simulink library "Lib_EMTAT"  (R2021b)
settings: Solver=VariableStepAuto  StartTime=0.0  StopTime=10.0  RelTol=1e-3
undefined symbols (not defined in the file or in its folder): A_M, B_M, Cj, component_degradation_input, Cs, E0_M, f_sw, K_M, MWS, Q_M, Q_rr, r_c, r_D, R_M, Rj, Ru, SNR_DX_M, SNR_IC_M, SNR_Mn_M, SNR_Mx_M, SOC_Init_M, u_ce0, u_D0
libraries: $bdroot x82, simulink x23, Lib_Dyn_StateSpace_EMTAT x3, PB_Library_Master_Working x1
(part 6 of 7)

== system Lib_EMTAT/Components/Physics-Based/Motor /Torque Saturation Logic ==
  note: Needs: P_m_max, T_ref_max
  T_ref_in : Inport
  S : Inport  Port=2
  Abs : Abs
  Constant1 : Constant  Value=P_out_max
  Display : Display
  Display1 : Display
  Display2 : Display
  Divide : Product  Inputs=*/
  Product : Product
  Sat in ft-lbs : Saturate  UpperLimit=T_nom  LowerLimit=-T_nom
  Switch : Switch  Criteria=u2 > Threshold  Threshold=P_out_max
  ft-lbs to Nm : Gain  Gain=1.3558
  ft-lbs to Nm1 : Gain  Gain=1.3558
  T_ref_sat : Outport  VectorParamsAs1DForOutWhenUnconnected=off
  wires:
  T_ref_in/1 -> Sat in ft-lbs/1, ft-lbs to Nm/1  "ft-lbs"
  Constant1/1 -> Display/1, Divide/1  "W"
  S/1 -> Product/2, Divide/2
  Sat in ft-lbs/1 -> ft-lbs to Nm1/1
  Product/1 -> Abs/1  "W"
  Switch/1 -> T_ref_sat/1
  ft-lbs to Nm/1 -> Product/1
  ft-lbs to Nm1/1 -> Switch/3, Display1/1  "Nm"
  Abs/1 -> Display2/1, Switch/2
  Divide/1 -> Switch/1  "Nm"

== system Lib_EMTAT/Components/Physics-Based/Motor /Vdq ==
  Id : Inport
  w_elec : Inport  Port=2
  Iq : Inport  Port=3
  Res_DF : Inport  Port=4
  Flux_DF : Inport  Port=5
  Divide : Product  Inputs=/*
  Divide1 : Product  Inputs=*/
  Gain : Gain  Gain=R_s
  Gain1 : Gain  Gain=R_s
  Gain2 : Gain  Gain=L_s
  Gain3 : Gain  Gain=flux_m
  Product : Product
  Product1 : Product
  Product2 : Product
  Subtract : Sum  Inputs=+-
  Sum : Sum  Inputs=+++
  Vd : Outport  VectorParamsAs1DForOutWhenUnconnected=off
  Vq : Outport  Port=2  VectorParamsAs1DForOutWhenUnconnected=off
  wires:
  Id/1 -> Product1/1, Gain/1
  Iq/1 -> Gain1/1, Product/2
  w_elec/1 -> Gain3/1, Gain2/1
  Gain2/1 -> Product/1, Product1/2
  Product/1 -> Subtract/2
  Subtract/1 -> Vd/1
  Product1/1 -> Sum/1
  Sum/1 -> Vq/1
  Gain3/1 -> Product2/1
  Product2/1 -> Sum/3
  Flux_DF/1 -> Product2/2
  Divide/1 -> Subtract/1
  Gain/1 -> Divide/2
  Res_DF/1 -> Divide/1, Divide1/2
  Divide1/1 -> Sum/2
  Gain1/1 -> Divide1/1

== system Lib_EMTAT/Components/Physics-Based/Motor /Vs ==
  Vd : Inport
  Vq : Inport  Port=2
  Add : Sum
  Square : Math  Operator=square  SignedPower=on  SaturateOnIntegerOverflow=on
  Square Root : Sqrt  SaturateOnIntegerOverflow=on
  Square1 : Math  Operator=square  SignedPower=on  SaturateOnIntegerOverflow=on
  Vs : Outport  VectorParamsAs1DForOutWhenUnconnected=off
  wires:
  Vq/1 -> Square/1
  Vd/1 -> Square1/1
  Square1/1 -> Add/1
  Square/1 -> Add/2
  Add/1 -> Square Root/1
  Square Root/1 -> Vs/1

== system Lib_EMTAT/Components/Physics-Based/Rectifier/Diode Conduction Losses1 ==
  note: update with gradual degredation term later
  note: the aDF must increase u_D_M
  note: You need to read from graphs:
      |
      | -U_ce0
      | -Rc=dU_ce/dI_c (linear)
      | -U_D0
      | -R_D=dU_D/dI_D (linear)
  I_M : Inport
  PF : Inport  Port=2
  m : Inport  Port=3
  T : Inport  Port=4
  1-D Lookup Table r_D : Lookup_n-D  NumberOfTableDimensions=1  BreakpointsForDimension1=T_M  Table=R_D_M  InternalRulePriority=Speed  RndMeth=Simplest  InputSameDT=on
  1-D Lookup Table u_D0 : Lookup_n-D  NumberOfTableDimensions=1  BreakpointsForDimension1=T_M  Table=u_D_M  InternalRulePriority=Speed  RndMeth=Simplest  InputSameDT=on
  Constant : Constant  Value=1/(2*pi)
  Constant1 : Constant  Value=1/8
  Gain : Gain  Commented=on  Gain=u_D0
  Gain1 : Gain  Gain=1/8
  Gain2 : Gain  Commented=on  Gain=r_D
  Gain3 : Gain  Gain=1/(3*pi)
  Product{,1..4} (5 alike) : Product
  Square : Math  Operator=square  SignedPower=on  SaturateOnIntegerOverflow=on
  Sum : Sum  Inputs=+-
  Sum2 : Sum
  Sum3 : Sum  Inputs=-+
  P_CD : Outport  VectorParamsAs1DForOutWhenUnconnected=off
  wires:
  1-D Lookup Table r_D/1 -> Product4/2
  1-D Lookup Table u_D0/1 -> Product3/2
  T/1 -> 1-D Lookup Table r_D/1, 1-D Lookup Table u_D0/1
  Sum3/1 -> Product2/2
  Constant1/1 -> Sum3/2
  Product4/1 -> Product2/1
  Gain3/1 -> Sum3/1
  Square/1 -> Product4/1
  Sum/1 -> Product/1
  Product1/1 -> Gain1/1, Gain3/1
  Gain1/1 -> Sum/2
  m/1 -> Product1/2
  PF/1 -> Product1/1
  Constant/1 -> Sum/1
  Product3/1 -> Square/1, Product/2
  I_M/1 -> Product3/1  "I_M"
  Sum2/1 -> P_CD/1
  Product2/1 -> Sum2/2
  Product/1 -> Sum2/1

== system Lib_EMTAT/Components/Physics-Based/Rectifier/IGBT Conduction Losses1 ==
  note: You need to read from graphs:
      |
      | -U_ce0
      | -Rc=dU_ce/dI_c (linear)
      | -U_D0
      | -R_D=dU_D/dI_D (linear)
  I_M : Inport
  PF : Inport  Port=2
  m : Inport  Port=3
  T : Inport  Port=4
  1-D Lookup Table r_c : Lookup_n-D  NumberOfTableDimensions=1  BreakpointsForDimension1=T_M  Table=R_c_M  InternalRulePriority=Speed  RndMeth=Simplest  InputSameDT=on
  1-D Lookup Table u_ce0 : Lookup_n-D  NumberOfTableDimensions=1  BreakpointsForDimension1=T_M  Table=u_ce0_M  InternalRulePriority=Speed  RndMeth=Simplest  InputSameDT=on
  Constant : Constant  Value=1/(2*pi)
  Constant1 : Constant  Value=1/8
  Gain : Gain  Commented=on  Gain=u_ce0
  Gain1 : Gain  Gain=1/8
  Gain2 : Gain  Commented=on  Gain=r_c
  Gain3 : Gain  Gain=1/(3*pi)
  Product{,1..4} (5 alike) : Product
  Square : Math  Operator=square  SignedPower=on  SaturateOnIntegerOverflow=on
  Sum : Sum
  Sum2 : Sum
  Sum3 : Sum
  P_CT : Outport  VectorParamsAs1DForOutWhenUnconnected=off
  wires:
  1-D Lookup Table r_c/1 -> Product4/2
  1-D Lookup Table u_ce0/1 -> Product3/2
  T/1 -> 1-D Lookup Table r_c/1, 1-D Lookup Table u_ce0/1
  Sum3/1 -> Product2/2
  Constant1/1 -> Sum3/2
  Product4/1 -> Product2/1
  Gain3/1 -> Sum3/1
  Square/1 -> Product4/1
  Sum/1 -> Product/1
  Product1/1 -> Gain1/1, Gain3/1
  Gain1/1 -> Sum/2
  m/1 -> Product1/2
  PF/1 -> Product1/1
  Constant/1 -> Sum/1
  Product3/1 -> Square/1, Product/2
  I_M/1 -> Product3/1  "I_M"
  Sum2/1 -> P_CT/1
  Product2/1 -> Sum2/2
  Product/1 -> Sum2/1

== system Lib_EMTAT/Components/Physics-Based/Rectifier/IGBT Switching Losses1 ==
  note: the aDF must increase E1_M
  note: update with gradual degredation term later
  I_ce : Inport
  T : Inport  Port=2
  1-D Lookup Table E0 : Lookup_n-D  NumberOfTableDimensions=1  BreakpointsForDimension1=T_M  Table=E0_M  InternalRulePriority=Speed  RndMeth=Simplest  InputSameDT=on
  1-D Lookup Table E1 : Lookup_n-D  NumberOfTableDimensions=1  BreakpointsForDimension1=T_M  Table=E1_M  InternalRulePriority=Speed  RndMeth=Simplest  InputSameDT=on
  Add : Sum
  Constant : Constant  Value=f_sw_M
  Constant1 : Constant
  Divide : Product  Inputs=*/
  Product : Product
  Product1 : Product
  P_ST : Outport  VectorParamsAs1DForOutWhenUnconnected=off
  wires:
  Product/1 -> P_ST/1
  Add/1 -> Product/1
  I_ce/1 -> Product1/1
  1-D Lookup Table E0/1 -> Add/1
  Product1/1 -> Add/2
  T/1 -> 1-D Lookup Table E0/1, 1-D Lookup Table E1/1
  1-D Lookup Table E1/1 -> Product1/2
  Constant/1 -> Divide/1
  Divide/1 -> Product/2
  Constant1/1 -> Divide/2

== system Lib_EMTAT/Components/Physics-Based/Rectifier/I_Ripple1 ==
  note: update with gradual degredation term later
  V_batt : Inport
  "V_M " : Inport  Port=2
  Constant : Constant  Value=L_s_M
  Constant1 : Constant
  Divide : Product  Inputs=*/
  Divide1 : Product  Inputs=*/
  Gain : Gain  Gain=sqrt(2)
  Gain1 : Gain  Gain=2
  Gain2 : Gain  Gain=f_sw_M
  Product : Product
  Product1 : Product
  Subtract : Sum  Inputs=+-
  I_Rip : Outport  VectorParamsAs1DForOutWhenUnconnected=off
  wires:
  Divide/1 -> I_Rip/1
  Product1/1 -> Gain2/1
  Gain1/1 -> Product1/2
  Constant/1 -> Gain1/1
  Product/1 -> Divide/1
  Subtract/1 -> Product/1
  V_batt/1 -> Product1/1, Subtract/1
  Gain/1 -> Subtract/2
  "V_M "/1 -> Gain/1, Product/2
  Gain2/1 -> Divide1/1
  Constant1/1 -> Divide1/2
  Divide1/1 -> Divide/2

== system Lib_EMTAT/Components/Physics-Based/Rectifier/P_out_gen ==
  I (DC) : Inport
  V_s (DC) : Inport  Port=2
  PF : Inport  Port=3
  Display : Display
  Gain : Gain  Commented=through  Gain=sqrt(3)
  PowerFactor StandIn : Constant
  Product : Product  Inputs=3
  P_out_gen : Outport  VectorParamsAs1DForOutWhenUnconnected=off
  wires:
  PowerFactor StandIn/1 -> Product/3
  Product/1 -> Gain/1
  Gain/1 -> P_out_gen/1
  V_s (DC)/1 -> Product/1
  PF/1 -> Display/1
  I (DC)/1 -> Product/2

== system Lib_EMTAT/Components/Physics-Based/Rectifier/mVal ==
  V_s : Inport
  V_batt : Inport  Port=2
  Divide : Product  Inputs=*/
  Gain : Gain  Gain=sqrt(2)
  m : Outport  VectorParamsAs1DForOutWhenUnconnected=off
  wires:
  V_batt/1 -> Divide/2
  Gain/1 -> Divide/1
  V_s/1 -> Gain/1
  Divide/1 -> m/1

== system Lib_EMTAT/Components/Power Flow/AC-AC Transformer/Compensate for Divide By Zero ==
  note: If Vin is not equal to zero, use its value.
      | If Vin is equal to zero, it will calculate a nan value for Iin. Set Iin to zero.
  P_AC_1 : Inport
  V_LN_rms_1 : Inport  Port=2
  Fix Divide By Zero. : Subsystem
  I_L_rms_1 : Outport
  wires:
  V_LN_rms_1/1 -> Fix Divide By Zero./1(V_LN_rms_1)
  P_AC_1/1 -> Fix Divide By Zero./2(P_AC_1)
  Fix Divide By Zero./1(I_L_rms_1) -> I_L_rms_1/1

== system Lib_EMTAT/Components/Power Flow/AC-AC Transformer/Direction Determination ==
  P_AC_2 : Inport
  Ploss : Inport  Port=2
  Add1 : Sum
  Switch : Switch  Criteria=u2 ~= 0
  P_AC_1 : Outport
  wires:
  Add1/1 -> Switch/1
  Switch/1 -> P_AC_1/1
  P_AC_2/1 -> Switch/2, Switch/3, Add1/2
  Ploss/1 -> Add1/1

== system Lib_EMTAT/Components/Power Flow/AC-AC Transformer/Efficiency ==
  P_AC_2 : Inport
  P_AC_1 : Inport  Port=2
  Abs : Abs
  Abs1 : Abs
  Fix Divide By Zero. : Subsystem
  Fix Divide By Zero.1 : Subsystem
  GreaterThan : RelationalOperator  OutDataTypeStr=boolean  RndMeth=Simplest
  Switch : Switch  Criteria=u2 > Threshold
  Eff : Outport
  wires:
  Switch/1 -> Eff/1
  GreaterThan/1 -> Switch/2
  Abs1/1 -> Fix Divide By Zero.1/2(abs(P_AC_2)), Fix Divide By Zero./1(abs(P_AC_2)), GreaterThan/2
  P_AC_1/1 -> Abs/1
  P_AC_2/1 -> Abs1/1
  Abs/1 -> Fix Divide By Zero.1/1(abs(P_AC_1)), Fix Divide By Zero./2(abs(P_AC_1)), GreaterThan/1
  Fix Divide By Zero./1(Eff) -> Switch/3
  Fix Divide By Zero.1/1(Eff) -> Switch/1

== system Lib_EMTAT/Components/Power Flow/AC-AC Transformer/Failure Determination ==
  Fail? : Inport
  Compare To Constant : simulink/Logic and Bit Operations/Compare To Constant  relop===  const=1  OutDataTypeStr=boolean
  Compare To Constant1 : simulink/Logic and Bit Operations/Compare To Constant  relop===  const=2  OutDataTypeStr=boolean
  Data Type Conversion : DataTypeConversion  OutDataTypeStr=double
  Data Type Conversion1 : DataTypeConversion  OutDataTypeStr=double
  Failure Mode : Constant  Value=FM
  Logical Operator : Logic  AllPortsSameDT=off  OutDataTypeStr=boolean
  Logical Operator1 : Logic  AllPortsSameDT=off  OutDataTypeStr=boolean
  OCFail : Outport
  DegFail : Outport  Port=2
  wires:
  Failure Mode/1 -> Compare To Constant1/1, Compare To Constant/1
  Compare To Constant/1 -> Logical Operator/1
  Logical Operator/1 -> Data Type Conversion/1
  Compare To Constant1/1 -> Logical Operator1/1
  Logical Operator1/1 -> Data Type Conversion1/1
  Fail?/1 -> Logical Operator1/2, Logical Operator/2
  Data Type Conversion1/1 -> DegFail/1
  Data Type Conversion/1 -> OCFail/1

== system Lib_EMTAT/Components/Power Flow/AC-AC Transformer/Open Circuit Failure - DC Current ==
  Failed? : Inport
  I_L_rms_1 : Inport  Port=2
  Constant : Constant  Value=0
  IsInf : RelationalOperator  Operator=isInf  OutDataTypeStr=boolean  RndMeth=Simplest
  IsNaN : RelationalOperator  Operator=isNaN  OutDataTypeStr=boolean  RndMeth=Simplest
  Logical Operator : Logic  Operator=OR  Inputs=3  AllPortsSameDT=off  OutDataTypeStr=boolean
  Switch : Switch  Criteria=u2 > Threshold
  "I_L_rms_1 " : Outport
  wires:
  Failed?/1 -> Logical Operator/1
  Constant/1 -> Switch/1
  I_L_rms_1/1 -> IsNaN/1, IsInf/1, Switch/3
  Switch/1 -> "I_L_rms_1 "/1
  Logical Operator/1 -> Switch/2
  IsNaN/1 -> Logical Operator/2
  IsInf/1 -> Logical Operator/3

== system Lib_EMTAT/Components/Power Flow/AC-AC Transformer/Open Circuit Failure - Line to Neutral Voltage ==
  Failed? : Inport
  V_LN_rms_2 : Inport  Port=2
  Constant : Constant  Value=0
  IsInf : RelationalOperator  Operator=isInf  OutDataTypeStr=boolean  RndMeth=Simplest
  IsNaN : RelationalOperator  Operator=isNaN  OutDataTypeStr=boolean  RndMeth=Simplest
  Logical Operator : Logic  Operator=OR  Inputs=3  AllPortsSameDT=off  OutDataTypeStr=boolean
  Switch : Switch  Criteria=u2 > Threshold
  "V_LN_rms_2 " : Outport
  wires:
  IsInf/1 -> Logical Operator/3
  IsNaN/1 -> Logical Operator/2
  Logical Operator/1 -> Switch/2
  Switch/1 -> "V_LN_rms_2 "/1
  V_LN_rms_2/1 -> Switch/3, IsInf/1, IsNaN/1
  Constant/1 -> Switch/1
  Failed?/1 -> Logical Operator/1

== system Lib_EMTAT/Components/Power Flow/AC-AC Transformer/Open Circuit// Degradation Failure ==
  Ploss : Inport
  DegFail? : Inport  Port=2
  OCFail? : Inport  Port=3
  Deg : Inport  Port=4
  Constant : Constant  Value=0
  Constant1 : Constant  Value=Plosslim
  Divide : Product  Inputs=**
  "If degradation failure, add to Ploss." : Switch  Criteria=u2 > Threshold
  "If open circuit failure, set Ploss = 0." : Switch  Criteria=u2 > Threshold
  Sum1 : Sum  Inputs=++|
  "Ploss " : Outport
  wires:
  DegFail?/1 -> "If degradation failure, add to Ploss."/2
  "If degradation failure, add to Ploss."/1 -> "If open circuit failure, set Ploss = 0."/3
  Ploss/1 -> Sum1/2, "If degradation failure, add to Ploss."/3
  Sum1/1 -> "If degradation failure, add to Ploss."/1
  Deg/1 -> Divide/2
  "If open circuit failure, set Ploss = 0."/1 -> "Ploss "/1
  OCFail?/1 -> "If open circuit failure, set Ploss = 0."/2
  Constant/1 -> "If open circuit failure, set Ploss = 0."/1
  Constant1/1 -> Divide/1
  Divide/1 -> Sum1/1

== system Lib_EMTAT/Components/Power Flow/AC-AC Transformer/Power Loss ==
  V_LN_rms_1 : Inport
  I_L_rms_2 : Inport  Port=2
  2-D Lookup Table : Lookup_n-D  BreakpointsForDimension1=X_C_VoltageAC1Vec_M  BreakpointsForDimension2=Y_C_CurrentAC2Vec_M  Table=T_C_PowLossArray_M  ExtrapMethod=Clip  UseLastTableValue=on  InternalRulePriority=Speed  RndMeth=Simplest  InputSameDT=on
      settings: InputPortMap=u0,u1
  Abs : Abs
  Abs1 : Abs
  Saturation : Saturate  UpperLimit=inf  LowerLimit=0
  Ploss : Outport
  wires:
  V_LN_rms_1/1 -> Abs/1
  Abs/1 -> 2-D Lookup Table/1
  Abs1/1 -> 2-D Lookup Table/2
  I_L_rms_2/1 -> Abs1/1
  2-D Lookup Table/1 -> Saturation/1
  Saturation/1 -> Ploss/1

== system Lib_EMTAT/Components/Power Flow/AC-DC Rectifier/Compensate for Divide By Zero. ==
  note: If Vin is not equal to zero, use its value.
      | If Vin is equal to zero, it will calculate a nan value for Iin. Set Iin to zero.
  PEquivAC : Inport
  V_LN_rms : Inport  Port=2
  Fix Divide By Zero. : Subsystem
  I_L_rms : Outport
  wires:
  Fix Divide By Zero./1(I_L_rms) -> I_L_rms/1
  PEquivAC/1 -> Fix Divide By Zero./2(PEquivAC)
  V_LN_rms/1 -> Fix Divide By Zero./1(V_LN_rms)

== system Lib_EMTAT/Components/Power Flow/AC-DC Rectifier/Direction Determination ==
  P_DC : Inport
  Ploss : Inport  Port=2
  Add1 : Sum  Inputs=-+
  Switch : Switch  Criteria=u2 ~= 0
  PEquivAC : Outport
  wires:
  P_DC/1 -> Switch/3, Switch/2, Add1/2
  Ploss/1 -> Add1/1
  Add1/1 -> Switch/1
  Switch/1 -> PEquivAC/1

== system Lib_EMTAT/Components/Power Flow/AC-DC Rectifier/Efficiency1 ==
  P_AC : Inport
  P_DC : Inport  Port=2
  Abs : Abs
  Abs1 : Abs
  Fix Divide By Zero. : Subsystem
  Fix Divide By Zero.1 : Subsystem
  GreaterThan : RelationalOperator  OutDataTypeStr=boolean  RndMeth=Simplest
  Switch : Switch  Criteria=u2 > Threshold
  Eff : Outport
  wires:
  Switch/1 -> Eff/1
  GreaterThan/1 -> Switch/2
  Abs1/1 -> Fix Divide By Zero.1/2(abs(P_AC)), Fix Divide By Zero./1(abs(P_AC)), GreaterThan/2
  P_DC/1 -> Abs/1
  P_AC/1 -> Abs1/1
  Abs/1 -> Fix Divide By Zero.1/1(abs(P_DC)), Fix Divide By Zero./2(abs(P_DC)), GreaterThan/1
  Fix Divide By Zero./1(Eff) -> Switch/3
  Fix Divide By Zero.1/1(Eff) -> Switch/1

== system Lib_EMTAT/Components/Power Flow/AC-DC Rectifier/Failure Determination1 ==
  Fail? : Inport
  Compare To Constant : simulink/Logic and Bit Operations/Compare To Constant  relop===  const=1  OutDataTypeStr=boolean
  Compare To Constant1 : simulink/Logic and Bit Operations/Compare To Constant  relop===  const=2  OutDataTypeStr=boolean
  Data Type Conversion : DataTypeConversion  OutDataTypeStr=double
  Data Type Conversion1 : DataTypeConversion  OutDataTypeStr=double
  Failure Mode : Constant  Value=FM
  Logical Operator : Logic  AllPortsSameDT=off  OutDataTypeStr=boolean
  Logical Operator1 : Logic  AllPortsSameDT=off  OutDataTypeStr=boolean
  OCFail : Outport
  DegFail : Outport  Port=2
  wires:
  Failure Mode/1 -> Compare To Constant1/1, Compare To Constant/1
  Compare To Constant/1 -> Logical Operator/1
  Logical Operator/1 -> Data Type Conversion/1
  Compare To Constant1/1 -> Logical Operator1/1
  Logical Operator1/1 -> Data Type Conversion1/1
  Fail?/1 -> Logical Operator1/2, Logical Operator/2
  Data Type Conversion1/1 -> DegFail/1
  Data Type Conversion/1 -> OCFail/1

== system Lib_EMTAT/Components/Power Flow/AC-DC Rectifier/Open Circuit Failure - DC Voltage ==
  Failed? : Inport
  V_DC : Inport  Port=2
  Constant : Constant  Value=0
  IsInf : RelationalOperator  Operator=isInf  OutDataTypeStr=boolean  RndMeth=Simplest
  IsNaN : RelationalOperator  Operator=isNaN  OutDataTypeStr=boolean  RndMeth=Simplest
  Logical Operator : Logic  Operator=OR  Inputs=3  AllPortsSameDT=off  OutDataTypeStr=boolean
  Switch : Switch  Criteria=u2 > Threshold
  "V_DC " : Outport
  wires:
  Failed?/1 -> Logical Operator/1
  Constant/1 -> Switch/1
  V_DC/1 -> IsNaN/1, IsInf/1, Switch/3
  Switch/1 -> "V_DC "/1
  Logical Operator/1 -> Switch/2
  IsNaN/1 -> Logical Operator/2
  IsInf/1 -> Logical Operator/3

== system Lib_EMTAT/Components/Power Flow/AC-DC Rectifier/Open Circuit// Degradation Failure ==
  Ploss : Inport
  DegFail? : Inport  Port=2
  OCFail? : Inport  Port=3
  Deg : Inport  Port=4
  Constant : Constant  Value=0
  Constant1 : Constant  Value=Plosslim
  Divide : Product  Inputs=**
  "If degradation failure, add to Ploss." : Switch  Criteria=u2 > Threshold
  "If open circuit failure, set Ploss = 0." : Switch  Criteria=u2 > Threshold
  Sum1 : Sum  Inputs=++|
  "Ploss " : Outport
  wires:
  Divide/1 -> Sum1/1
  Constant1/1 -> Divide/1
  Constant/1 -> "If open circuit failure, set Ploss = 0."/1
  OCFail?/1 -> "If open circuit failure, set Ploss = 0."/2
  "If open circuit failure, set Ploss = 0."/1 -> "Ploss "/1
  Deg/1 -> Divide/2
  Sum1/1 -> "If degradation failure, add to Ploss."/1
  Ploss/1 -> "If degradation failure, add to Ploss."/3, Sum1/2
  "If degradation failure, add to Ploss."/1 -> "If open circuit failure, set Ploss = 0."/3
  DegFail?/1 -> "If degradation failure, add to Ploss."/2

== system Lib_EMTAT/Components/Power Flow/AC-DC Rectifier/Power Loss ==
  V_DC : Inport
  I_L_rms : Inport  Port=2
  2-D Lookup Table : Lookup_n-D  BreakpointsForDimension1=X_C_VoltageInVec_M  BreakpointsForDimension2=Y_C_RMSCurrentOutVec_M  Table=T_C_PowLossArray_M  ExtrapMethod=Clip  UseLastTableValue=on  InternalRulePriority=Speed  RndMeth=Simplest  InputSameDT=on
      settings: InputPortMap=u0,u1
  Abs : Abs
  Abs1 : Abs
  Saturation : Saturate  UpperLimit=inf  LowerLimit=0
  Ploss : Outport
  wires:
  V_DC/1 -> Abs/1
  Abs/1 -> 2-D Lookup Table/1
  Abs1/1 -> 2-D Lookup Table/2
  I_L_rms/1 -> Abs1/1
  2-D Lookup Table/1 -> Saturation/1
  Saturation/1 -> Ploss/1

== system Lib_EMTAT/Components/Power Flow/Cable/Failure Determination ==
  Fail? : Inport
  OCFail : Outport
  wires:
  Fail?/1 -> OCFail/1

== system Lib_EMTAT/Components/Power Flow/Cable/Fix Zero Voltage Problem ==
  note: If Vin is not equal to zero, pass Vout.
      | If Vin is equal to zero, set Vout to zero. This has to be done because a Vin of 0 would take an efficiency hit and produce a negative Vout.
      | In reality, a zero voltage does not take an efficiency hit.
  "Vout " : Inport
  Vin : Inport  Port=2
  Constant : Constant  Value=0
  Switch : Switch  Criteria=u2 ~= 0
  Vout : Outport
  wires:
  Vin/1 -> Switch/2
  "Vout "/1 -> Switch/1
  Constant/1 -> Switch/3
  Switch/1 -> Vout/1

== system Lib_EMTAT/Components/Power Flow/Cable/Open Circuit Failure - Current ==
  Failed? : Inport
  Iin/Iout : Inport  Port=2
  Constant : Constant  Value=0
  IsInf : RelationalOperator  Operator=isInf  OutDataTypeStr=boolean  RndMeth=Simplest
  IsNaN : RelationalOperator  Operator=isNaN  OutDataTypeStr=boolean  RndMeth=Simplest
  Logical Operator : Logic  Operator=OR  Inputs=3  AllPortsSameDT=off  OutDataTypeStr=boolean
  Switch : Switch  Criteria=u2 > Threshold
  "Iin/Iout " : Outport
  wires:
  Failed?/1 -> Logical Operator/1
  Constant/1 -> Switch/1
  Iin/Iout/1 -> IsNaN/1, IsInf/1, Switch/3
  Switch/1 -> "Iin/Iout "/1
  Logical Operator/1 -> Switch/2
  IsNaN/1 -> Logical Operator/2
  IsInf/1 -> Logical Operator/3

== system Lib_EMTAT/Components/Power Flow/Cable/Open Circuit Failure - Voltage ==
  Failed? : Inport
  Vout : Inport  Port=2
  Constant : Constant  Value=0
  IsInf : RelationalOperator  Operator=isInf  OutDataTypeStr=boolean  RndMeth=Simplest
  IsNaN : RelationalOperator  Operator=isNaN  OutDataTypeStr=boolean  RndMeth=Simplest
  Logical Operator : Logic  Operator=OR  Inputs=3  AllPortsSameDT=off  OutDataTypeStr=boolean
  Switch : Switch  Criteria=u2 > Threshold
  "Vout " : Outport
  wires:
  IsInf/1 -> Logical Operator/3
  IsNaN/1 -> Logical Operator/2
  Logical Operator/1 -> Switch/2
  Switch/1 -> "Vout "/1
  Vout/1 -> Switch/3, IsInf/1, IsNaN/1
  Constant/1 -> Switch/1
  Failed?/1 -> Logical Operator/1

== system Lib_EMTAT/Components/Power Flow/DC-AC Inverter/Compensate for Divide By Zero ==
  note: If Vin is not equal to zero, use its value.
      | If Vin is equal to zero, it will calculate a nan value for Iin. Set Iin to zero.
  PEquivDC : Inport
  V_DC : Inport  Port=2
  Fix Divide By Zero. : Subsystem
  I_DC : Outport
  wires:
  Fix Divide By Zero./1(I_DC) -> I_DC/1
  PEquivDC/1 -> Fix Divide By Zero./2(PEquivDC)
  V_DC/1 -> Fix Divide By Zero./1(V_DC)

== system Lib_EMTAT/Components/Power Flow/DC-AC Inverter/Direction Determination ==
  P_AC : Inport
  Ploss : Inport  Port=2
  Add1 : Sum
  Switch : Switch  Criteria=u2 ~= 0
  PEquivDC : Outport
  wires:
  Add1/1 -> Switch/1
  Ploss/1 -> Add1/1
  P_AC/1 -> Switch/3, Switch/2, Add1/2
  Switch/1 -> PEquivDC/1

== system Lib_EMTAT/Components/Power Flow/DC-AC Inverter/Open Circuit Failure - DC Current ==
  Failed? : Inport
  I_DC : Inport  Port=2
  Constant : Constant  Value=0
  IsInf : RelationalOperator  Operator=isInf  OutDataTypeStr=boolean  RndMeth=Simplest
  IsNaN : RelationalOperator  Operator=isNaN  OutDataTypeStr=boolean  RndMeth=Simplest
  Logical Operator : Logic  Operator=OR  Inputs=3  AllPortsSameDT=off  OutDataTypeStr=boolean
  Switch : Switch  Criteria=u2 > Threshold
  "I_DC " : Outport
  wires:
  IsInf/1 -> Logical Operator/3
  IsNaN/1 -> Logical Operator/2
  Logical Operator/1 -> Switch/2
  Switch/1 -> "I_DC "/1
  I_DC/1 -> Switch/3, IsInf/1, IsNaN/1
  Constant/1 -> Switch/1
  Failed?/1 -> Logical Operator/1

== system Lib_EMTAT/Components/Power Flow/DC-AC Inverter/Open Circuit Failure - Line to Neutral Voltage ==
  Failed? : Inport
  V_LN_rms : Inport  Port=2
  Constant : Constant  Value=0
  IsInf : RelationalOperator  Operator=isInf  OutDataTypeStr=boolean  RndMeth=Simplest
  IsNaN : RelationalOperator  Operator=isNaN  OutDataTypeStr=boolean  RndMeth=Simplest
  Logical Operator : Logic  Operator=OR  Inputs=3  AllPortsSameDT=off  OutDataTypeStr=boolean
  Switch : Switch  Criteria=u2 > Threshold
  "V_LN_rms " : Outport
  wires:
  Failed?/1 -> Logical Operator/1
  Constant/1 -> Switch/1
  V_LN_rms/1 -> IsNaN/1, IsInf/1, Switch/3
  Switch/1 -> "V_LN_rms "/1
  Logical Operator/1 -> Switch/2
  IsNaN/1 -> Logical Operator/2
  IsInf/1 -> Logical Operator/3

== system Lib_EMTAT/Components/Power Flow/DC-AC Inverter/Open Circuit// Degradation Failure ==
  Ploss : Inport
  DegFail? : Inport  Port=2
  OCFail? : Inport  Port=3
  Deg : Inport  Port=4
  Constant : Constant  Value=0
  Constant1 : Constant  Value=Plosslim
  Divide : Product  Inputs=**
  "If degradation failure, add to Ploss." : Switch  Criteria=u2 > Threshold
  "If open circuit failure, set Ploss = 0." : Switch  Criteria=u2 > Threshold
  Sum1 : Sum  Inputs=++|
  "Ploss " : Outport
  wires:
  Divide/1 -> Sum1/1
  Constant1/1 -> Divide/1
  Constant/1 -> "If open circuit failure, set Ploss = 0."/1
  OCFail?/1 -> "If open circuit failure, set Ploss = 0."/2
  "If open circuit failure, set Ploss = 0."/1 -> "Ploss "/1
  Deg/1 -> Divide/2
  Sum1/1 -> "If degradation failure, add to Ploss."/1
  Ploss/1 -> "If degradation failure, add to Ploss."/3, Sum1/2
  "If degradation failure, add to Ploss."/1 -> "If open circuit failure, set Ploss = 0."/3
  DegFail?/1 -> "If degradation failure, add to Ploss."/2

== system Lib_EMTAT/Components/Power Flow/DC-AC Inverter/Power Loss ==
  V_DC : Inport
  I_L_rms : Inport  Port=2
  2-D Lookup Table : Lookup_n-D  BreakpointsForDimension1=X_C_VoltageInVec_M  BreakpointsForDimension2=Y_C_RMSCurrentOutVec_M  Table=T_C_PowLossArray_M  ExtrapMethod=Clip  UseLastTableValue=on  InternalRulePriority=Speed  RndMeth=Simplest  InputSameDT=on
      settings: InputPortMap=u0,u1
  Abs : Abs
  Abs1 : Abs
  Saturation : Saturate  UpperLimit=inf  LowerLimit=0
  Ploss : Outport
  wires:
  Saturation/1 -> Ploss/1
  2-D Lookup Table/1 -> Saturation/1
  I_L_rms/1 -> Abs1/1
  Abs1/1 -> 2-D Lookup Table/2
  Abs/1 -> 2-D Lookup Table/1
  V_DC/1 -> Abs/1

== system Lib_EMTAT/Components/Power Flow/DC-DC Converter (Set Output Voltage)/Compensate for Divide By Zero ==
  note: If Vin is not equal to zero, use its value.
      | If Vin is equal to zero, it will calculate a nan value for Iin. Set Iin to zero.
  Pin : Inport
  Vin : Inport  Port=2
  Fix Divide By Zero. : Subsystem
  Iin : Outport
  wires:
  Fix Divide By Zero./1(Iin) -> Iin/1
  Pin/1 -> Fix Divide By Zero./2(Pin)
  Vin/1 -> Fix Divide By Zero./1(Vin)

== system Lib_EMTAT/Components/Power Flow/DC-DC Converter (Set Output Voltage)/Direction Determination ==
  Pout : Inport
  Ploss : Inport  Port=2
  Add1 : Sum
  Switch : Switch  Criteria=u2 ~= 0
  Pin : Outport
  wires:
  Switch/1 -> Pin/1
  Pout/1 -> Add1/2, Switch/2, Switch/3
  Ploss/1 -> Add1/1
  Add1/1 -> Switch/1

== system Lib_EMTAT/Components/Power Flow/DC-DC Converter (Set Output Voltage)/Efficiency ==
  Pout : Inport
  Pin : Inport  Port=2
  Abs : Abs
  Abs1 : Abs
  Fix Divide By Zero. : Subsystem
  Fix Divide By Zero.1 : Subsystem
  GreaterThan : RelationalOperator  OutDataTypeStr=boolean  RndMeth=Simplest
  Switch : Switch  Criteria=u2 > Threshold
  Eff : Outport
  wires:
  Fix Divide By Zero.1/1(Eff) -> Switch/1
  Fix Divide By Zero./1(Eff) -> Switch/3
  Abs/1 -> GreaterThan/1, Fix Divide By Zero./2(abs(Pin)), Fix Divide By Zero.1/1(abs(Pin))
  Pout/1 -> Abs1/1
  Pin/1 -> Abs/1
  Abs1/1 -> GreaterThan/2, Fix Divide By Zero./1(abs(Pout)), Fix Divide By Zero.1/2(abs(Pout))
  GreaterThan/1 -> Switch/2
  Switch/1 -> Eff/1

== system Lib_EMTAT/Components/Power Flow/DC-DC Converter (Set Output Voltage)/Failure Determination ==
  Fail? : Inport
  Compare To Constant : simulink/Logic and Bit Operations/Compare To Constant  relop===  const=1  OutDataTypeStr=boolean
  Compare To Constant1 : simulink/Logic and Bit Operations/Compare To Constant  relop===  const=2  OutDataTypeStr=boolean
  Data Type Conversion : DataTypeConversion  OutDataTypeStr=double
  Data Type Conversion1 : DataTypeConversion  OutDataTypeStr=double
  Failure Mode : Constant  Value=FM
  Logical Operator : Logic  AllPortsSameDT=off  OutDataTypeStr=boolean
  Logical Operator1 : Logic  AllPortsSameDT=off  OutDataTypeStr=boolean
  OCFail : Outport
  DegFail : Outport  Port=2
  wires:
  Data Type Conversion/1 -> OCFail/1
  Data Type Conversion1/1 -> DegFail/1
  Fail?/1 -> Logical Operator/2, Logical Operator1/2
  Logical Operator1/1 -> Data Type Conversion1/1
  Compare To Constant1/1 -> Logical Operator1/1
  Logical Operator/1 -> Data Type Conversion/1
  Compare To Constant/1 -> Logical Operator/1
  Failure Mode/1 -> Compare To Constant/1, Compare To Constant1/1

== system Lib_EMTAT/Components/Power Flow/DC-DC Converter (Set Output Voltage)/Open Circuit Failure - Input Current ==
  Failed? : Inport
  Iin : Inport  Port=2
  Constant : Constant  Value=0
  IsInf : RelationalOperator  Operator=isInf  OutDataTypeStr=boolean  RndMeth=Simplest
  IsNaN : RelationalOperator  Operator=isNaN  OutDataTypeStr=boolean  RndMeth=Simplest
  Logical Operator : Logic  Operator=OR  Inputs=3  AllPortsSameDT=off  OutDataTypeStr=boolean
  Switch : Switch  Criteria=u2 > Threshold
  "Iin  " : Outport
  wires:
  IsInf/1 -> Logical Operator/3
  IsNaN/1 -> Logical Operator/2
  Logical Operator/1 -> Switch/2
  Switch/1 -> "Iin  "/1
  Iin/1 -> Switch/3, IsInf/1, IsNaN/1
  Constant/1 -> Switch/1
  Failed?/1 -> Logical Operator/1

== system Lib_EMTAT/Components/Power Flow/DC-DC Converter (Set Output Voltage)/Open Circuit Failure - Output Voltage ==
  Failed? : Inport
  Vout : Inport  Port=2
  Constant : Constant  Value=0
  IsInf : RelationalOperator  Operator=isInf  OutDataTypeStr=boolean  RndMeth=Simplest
  IsNaN : RelationalOperator  Operator=isNaN  OutDataTypeStr=boolean  RndMeth=Simplest
  Logical Operator : Logic  Operator=OR  Inputs=3  AllPortsSameDT=off  OutDataTypeStr=boolean
  Switch : Switch  Criteria=u2 > Threshold
  "Vout   " : Outport
  wires:
  Failed?/1 -> Logical Operator/1
  Constant/1 -> Switch/1
  Vout/1 -> IsNaN/1, IsInf/1, Switch/3
  Switch/1 -> "Vout   "/1
  Logical Operator/1 -> Switch/2
  IsNaN/1 -> Logical Operator/2
  IsInf/1 -> Logical Operator/3

== system Lib_EMTAT/Components/Power Flow/DC-DC Converter (Set Output Voltage)/Open Circuit// Degradation Failure ==
  Ploss : Inport
  DegFail? : Inport  Port=2
  OCFail? : Inport  Port=3
  Deg : Inport  Port=4
  Constant : Constant  Value=0
  Constant1 : Constant  Value=Plosslim
  Divide : Product  Inputs=**
  "If degradation failure, add to Ploss." : Switch  Criteria=u2 > Threshold
  "If open circuit failure, set Ploss = 0." : Switch  Criteria=u2 > Threshold
  Sum1 : Sum  Inputs=++|
  "Ploss " : Outport
  wires:
  Divide/1 -> Sum1/1
  Constant1/1 -> Divide/1
  Constant/1 -> "If open circuit failure, set Ploss = 0."/1
  OCFail?/1 -> "If open circuit failure, set Ploss = 0."/2
  "If open circuit failure, set Ploss = 0."/1 -> "Ploss "/1
  Deg/1 -> Divide/2
  Sum1/1 -> "If degradation failure, add to Ploss."/1
  Ploss/1 -> "If degradation failure, add to Ploss."/3, Sum1/2
  "If degradation failure, add to Ploss."/1 -> "If open circuit failure, set Ploss = 0."/3
  DegFail?/1 -> "If degradation failure, add to Ploss."/2

== system Lib_EMTAT/Components/Power Flow/DC-DC Converter (Set Output Voltage)/Power Loss ==
  Vin : Inport
  Iout : Inport  Port=2
  2-D Lookup Table : Lookup_n-D  BreakpointsForDimension1=X_Vin_VoltageVec_M  BreakpointsForDimension2=Y_Iout_CurrentVec_M  Table=T_C_PlossArray_M  ExtrapMethod=Clip  UseLastTableValue=on  InternalRulePriority=Speed  RndMeth=Simplest  InputSameDT=on
      settings: InputPortMap=u0,u1
  Abs : Abs
  Abs1 : Abs
  Ploss : Outport
  wires:
  Vin/1 -> Abs/1
  Abs/1 -> 2-D Lookup Table/1
  Abs1/1 -> 2-D Lookup Table/2
  Iout/1 -> Abs1/1
  2-D Lookup Table/1 -> Ploss/1

== system Lib_EMTAT/Components/Power Flow/DC-DC Converter (Regulate Output Voltage)/Compensate for Divide By Zero ==
  note: If Vin is not equal to zero, use its value.
      | If Vin is equal to zero, it will calculate a nan value for Iin. Set Iin to zero.
  Pin : Inport
  Vin : Inport  Port=2
  Fix Divide By Zero. : Subsystem
  Iin : Outport
  wires:
  Vin/1 -> Fix Divide By Zero./1(Vin)
  Pin/1 -> Fix Divide By Zero./2(Pin)
  Fix Divide By Zero./1(Iin) -> Iin/1

== system Lib_EMTAT/Components/Power Flow/DC-DC Converter (Regulate Output Voltage)/Direction Determination ==
  Pout : Inport
  Ploss : Inport  Port=2
  Add1 : Sum
  Switch : Switch  Criteria=u2 ~= 0
  Pin : Outport
  wires:
  Add1/1 -> Switch/1
  Ploss/1 -> Add1/1
  Pout/1 -> Switch/3, Switch/2, Add1/2
  Switch/1 -> Pin/1

== system Lib_EMTAT/Components/Power Flow/DC-DC Converter (Regulate Output Voltage)/Efficiency ==
  Pout : Inport
  Pin : Inport  Port=2
  Abs : Abs
  Abs1 : Abs
  Fix Divide By Zero. : Subsystem
  Fix Divide By Zero.1 : Subsystem
  GreaterThan : RelationalOperator  OutDataTypeStr=boolean  RndMeth=Simplest
  Switch : Switch  Criteria=u2 > Threshold
  Eff : Outport
  wires:
  Switch/1 -> Eff/1
  GreaterThan/1 -> Switch/2
  Abs1/1 -> Fix Divide By Zero.1/2(abs(Pout)), Fix Divide By Zero./1(abs(Pout)), GreaterThan/2
  Pin/1 -> Abs/1
  Pout/1 -> Abs1/1
  Abs/1 -> Fix Divide By Zero.1/1(abs(Pin)), Fix Divide By Zero./2(abs(Pin)), GreaterThan/1
  Fix Divide By Zero./1(Eff) -> Switch/3
  Fix Divide By Zero.1/1(Eff) -> Switch/1

== system Lib_EMTAT/Components/Power Flow/DC-DC Converter (Regulate Output Voltage)/Failure Determination ==
  Fail? : Inport
  Compare To Constant : simulink/Logic and Bit Operations/Compare To Constant  relop===  const=1  OutDataTypeStr=boolean
  Compare To Constant1 : simulink/Logic and Bit Operations/Compare To Constant  relop===  const=2  OutDataTypeStr=boolean
  Data Type Conversion : DataTypeConversion  OutDataTypeStr=double
  Data Type Conversion1 : DataTypeConversion  OutDataTypeStr=double
  Failure Mode : Constant  Value=FM
  Logical Operator : Logic  AllPortsSameDT=off  OutDataTypeStr=boolean
  Logical Operator1 : Logic  AllPortsSameDT=off  OutDataTypeStr=boolean
  OCFail : Outport
  DegFail : Outport  Port=2
  wires:
  Failure Mode/1 -> Compare To Constant1/1, Compare To Constant/1
  Compare To Constant/1 -> Logical Operator/1
  Logical Operator/1 -> Data Type Conversion/1
  Compare To Constant1/1 -> Logical Operator1/1
  Logical Operator1/1 -> Data Type Conversion1/1
  Fail?/1 -> Logical Operator1/2, Logical Operator/2
  Data Type Conversion1/1 -> DegFail/1
  Data Type Conversion/1 -> OCFail/1

== system Lib_EMTAT/Components/Power Flow/DC-DC Converter (Regulate Output Voltage)/Open Circuit Failure - Input Current ==
  Failed? : Inport
  Iin : Inport  Port=2
  Constant : Constant  Value=0
  IsInf : RelationalOperator  Operator=isInf  OutDataTypeStr=boolean  RndMeth=Simplest
  IsNaN : RelationalOperator  Operator=isNaN  OutDataTypeStr=boolean  RndMeth=Simplest
  Logical Operator : Logic  Operator=OR  Inputs=3  AllPortsSameDT=off  OutDataTypeStr=boolean
  Switch : Switch  Criteria=u2 > Threshold
  "Iin  " : Outport
  wires:
  Failed?/1 -> Logical Operator/1
  Constant/1 -> Switch/1
  Iin/1 -> IsNaN/1, IsInf/1, Switch/3
  Switch/1 -> "Iin  "/1
  Logical Operator/1 -> Switch/2
  IsNaN/1 -> Logical Operator/2
  IsInf/1 -> Logical Operator/3

== system Lib_EMTAT/Components/Power Flow/DC-DC Converter (Regulate Output Voltage)/Open Circuit Failure - Output Voltage ==
  Failed? : Inport
  Vout : Inport  Port=2
  Constant : Constant  Value=0
  IsInf : RelationalOperator  Operator=isInf  OutDataTypeStr=boolean  RndMeth=Simplest
  IsNaN : RelationalOperator  Operator=isNaN  OutDataTypeStr=boolean  RndMeth=Simplest
  Logical Operator : Logic  Operator=OR  Inputs=3  AllPortsSameDT=off  OutDataTypeStr=boolean
  Switch : Switch  Criteria=u2 > Threshold
  "Vout   " : Outport
  wires:
  IsInf/1 -> Logical Operator/3
  IsNaN/1 -> Logical Operator/2
  Logical Operator/1 -> Switch/2
  Switch/1 -> "Vout   "/1
  Vout/1 -> Switch/3, IsInf/1, IsNaN/1
  Constant/1 -> Switch/1
  Failed?/1 -> Logical Operator/1

== system Lib_EMTAT/Components/Power Flow/DC-DC Converter (Regulate Output Voltage)/Open Circuit// Degradation Failure ==
  Ploss : Inport
  DegFail? : Inport  Port=2
  OCFail? : Inport  Port=3
  Deg : Inport  Port=4
  Constant : Constant  Value=0
  Constant1 : Constant  Value=Plosslim
  Divide : Product  Inputs=**
  "If degradation failure, add to Ploss." : Switch  Criteria=u2 > Threshold
  "If open circuit failure, set Ploss = 0." : Switch  Criteria=u2 > Threshold
  Sum1 : Sum  Inputs=++|
  "Ploss " : Outport
  wires:
  DegFail?/1 -> "If degradation failure, add to Ploss."/2
  "If degradation failure, add to Ploss."/1 -> "If open circuit failure, set Ploss = 0."/3
  Ploss/1 -> Sum1/2, "If degradation failure, add to Ploss."/3
  Sum1/1 -> "If degradation failure, add to Ploss."/1
  Deg/1 -> Divide/2
  "If open circuit failure, set Ploss = 0."/1 -> "Ploss "/1
  OCFail?/1 -> "If open circuit failure, set Ploss = 0."/2
  Constant/1 -> "If open circuit failure, set Ploss = 0."/1
  Constant1/1 -> Divide/1
  Divide/1 -> Sum1/1

== system Lib_EMTAT/Components/Power Flow/DC-DC Converter (Regulate Output Voltage)/Power Loss ==
  Vin : Inport
  Iout : Inport  Port=2
  2-D Lookup Table : Lookup_n-D  BreakpointsForDimension1=X_Vin_VoltageVec_M  BreakpointsForDimension2=Y_Iout_CurrentVec_M  Table=T_C_PlossArray_M  ExtrapMethod=Clip  UseLastTableValue=on  InternalRulePriority=Speed  RndMeth=Simplest  InputSameDT=on
      settings: InputPortMap=u0,u1
  Abs : Abs
  Abs1 : Abs
  Ploss : Outport
  wires:
  2-D Lookup Table/1 -> Ploss/1
  Iout/1 -> Abs1/1
  Abs1/1 -> 2-D Lookup Table/2
  Abs/1 -> 2-D Lookup Table/1
  Vin/1 -> Abs/1

== system Lib_EMTAT/Components/Power Flow/Energy Storage Device/SOC ==
  Energy (W-h) : Inport
  Divide : Product  Inputs=*/
  Gain : Gain  Gain=100
  Total Stored Energy (W-h) : Constant  Value=TSE
  SOC : Outport
  wires:
  Gain/1 -> SOC/1
  Divide/1 -> Gain/1
  Total Stored Energy (W-h)/1 -> Divide/2
  Energy (W-h)/1 -> Divide/1

== system Lib_EMTAT/Components/Power Flow/Energy Storage Device/Voltage, V to Energy, Wh ==
  V : Inport
  Gain2 : Gain  Gain=0.5*C
  J to Wh : Gain  Gain=0.000277778
  Square : Math  Operator=square  SaturateOnIntegerOverflow=on
  E : Outport
  wires:
  V/1 -> Square/1
  Gain2/1 -> J to Wh/1
  Square/1 -> Gain2/1
  J to Wh/1 -> E/1

== system Lib_EMTAT/Components/Power Flow/Energy Storage Device/Warnings ==
  SOC : Inport
  Compare To Constant : simulink/Logic and Bit Operations/Compare To Constant  relop=>  const=100  OutDataTypeStr=boolean
  Compare To Constant1 : simulink/Logic and Bit Operations/Compare To Constant  relop=<=  const=0  OutDataTypeStr=uint8
  Compare To Constant2 : simulink/Logic and Bit Operations/Compare To Constant  relop=<  const=2  OutDataTypeStr=boolean
  Logical Operator : Logic  AllPortsSameDT=off  OutDataTypeStr=boolean
  Memory : Memory
  SOC <= 0% : Subsystem
  SOC > 100% : Subsystem
  Sum : Sum  Inputs=|++
  wires:
  Logical Operator/1 -> SOC <= 0%/Trigger
  Compare To Constant2/1 -> Logical Operator/1
  Sum/1 -> Memory/1, Compare To Constant2/1
  Memory/1 -> Sum/2
  Compare To Constant1/1 -> Sum/1, Logical Operator/2
  Compare To Constant/1 -> SOC > 100%/Trigger
  SOC/1 -> Compare To Constant/1, Compare To Constant1/1

== system Lib_EMTAT/Components/Power Flow/Mechanical Shaft/Failure Determination ==
  Fail? : Inport
  SBFail : Outport
  wires:
  Fail?/1 -> SBFail/1

== system Lib_EMTAT/Components/Power Flow/Mechanical Shaft/Shaft Break Failure ==
  Failed? : Inport
  T : Inport  Port=2
  Constant : Constant  Value=0
  IsInf : RelationalOperator  Operator=isInf  OutDataTypeStr=boolean  RndMeth=Simplest
  IsNaN : RelationalOperator  Operator=isNaN  OutDataTypeStr=boolean  RndMeth=Simplest
  Logical Operator : Logic  Operator=OR  Inputs=3  AllPortsSameDT=off  OutDataTypeStr=boolean
  Switch : Switch  Criteria=u2 > Threshold
  "T " : Outport
  wires:
  Failed?/1 -> Logical Operator/1
  Constant/1 -> Switch/1
  T/1 -> IsNaN/1, IsInf/1, Switch/3
  Switch/1 -> "T "/1
  Logical Operator/1 -> Switch/2
  IsNaN/1 -> Logical Operator/2
  IsInf/1 -> Logical Operator/3

== system Lib_EMTAT/Components/Power Flow/Resistive Load Bank/Failure Determination ==
  Fail? : Inport
  OCFail : Outport
  wires:
  Fail?/1 -> OCFail/1

== system Lib_EMTAT/Components/Power Flow/Resistive Load Bank/Fix Divide By Zero. ==
  I^2 : Inport
  abs(Pset) : Inport  Port=2
  Constant : Constant  Value=0
  Divide1 : Product  Inputs=/*
  Switch : Switch  Criteria=u2 ~= 0
  R : Outport
  wires:
  Switch/1 -> R/1
  abs(Pset)/1 -> Divide1/2
  I^2/1 -> Switch/2, Divide1/1
  Divide1/1 -> Switch/1
  Constant/1 -> Switch/3

== system Lib_EMTAT/Components/Power Flow/Resistive Load Bank/Fix Divide By Zero.1 ==
  V : Inport
  Pset : Inport  Port=2
  Constant : Constant  Value=0
  Divide1 : Product  Inputs=/*
  Switch : Switch  Criteria=u2 ~= 0
  I : Outport
  wires:
  V/1 -> Switch/2, Divide1/1
  Pset/1 -> Divide1/2
  Switch/1 -> I/1
  Divide1/1 -> Switch/1
  Constant/1 -> Switch/3

== system Lib_EMTAT/Components/Power Flow/Resistive Load Bank/Open Circuit Failure - Line to Neutral Voltage ==
  Failed? : Inport
  I : Inport  Port=2
  Constant : Constant  Value=0
  IsInf : RelationalOperator  Operator=isInf  OutDataTypeStr=boolean  RndMeth=Simplest
  IsNaN : RelationalOperator  Operator=isNaN  OutDataTypeStr=boolean  RndMeth=Simplest
  Logical Operator : Logic  Operator=OR  Inputs=3  AllPortsSameDT=off  OutDataTypeStr=boolean
  Switch : Switch  Criteria=u2 > Threshold
  "I " : Outport
  wires:
  Failed?/1 -> Logical Operator/1
  Constant/1 -> Switch/1
  I/1 -> IsNaN/1, IsInf/1, Switch/3
  Switch/1 -> "I "/1
  Logical Operator/1 -> Switch/2
  IsNaN/1 -> Logical Operator/2
  IsInf/1 -> Logical Operator/3

== system Lib_EMTAT/Components/Power Flow/Three Phase Electric Machine (Sink)/Compensate for Divide By Zero ==
  note: If Vin is not equal to zero, use its value.
      | If Vin is equal to zero, it will calculate a nan value for Iin. Set Iin to zero.
  V_LN_rms : Inport
  PEquivElect : Inport  Port=2
  Fix Divide By Zero. : Subsystem
  I_L_rms : Outport
  wires:
  Fix Divide By Zero./1(I_L_rms) -> I_L_rms/1
  PEquivElect/1 -> Fix Divide By Zero./2(PEquivElect)
  V_LN_rms/1 -> Fix Divide By Zero./1(V_LN_rms)

== system Lib_EMTAT/Components/Power Flow/Three Phase Electric Machine (Sink)/Direction Determination ==
  PMech : Inport
  Eff : Inport  Port=2
  Divide : Product  Inputs=/*
  Divide1 : Product  Inputs=**
  Switch : Switch  Criteria=u2 > Threshold
  PEquivElect : Outport
  wires:
  Switch/1 -> PEquivElect/1
  Eff/1 -> Divide1/2, Divide/1
  Divide1/1 -> Switch/3
  Divide/1 -> Switch/1
  PMech/1 -> Switch/2, Divide/2, Divide1/1

== system Lib_EMTAT/Components/Power Flow/Three Phase Electric Machine (Sink)/Efficiency ==
  T : Inport
  N : Inport  Port=2
  2-D Lookup Table : Lookup_n-D  BreakpointsForDimension1=X_C_SpeedVec_M  BreakpointsForDimension2=Y_C_TorqueVec_M  Table=T_C_EffArray_M  ExtrapMethod=Clip  UseLastTableValue=on  InternalRulePriority=Speed  RndMeth=Simplest  InputSameDT=on
      settings: InputPortMap=u0,u1
  Abs : Abs
  Abs1 : Abs
  Eff : Outport
  wires:
  2-D Lookup Table/1 -> Eff/1
  N/1 -> Abs1/1
  Abs1/1 -> 2-D Lookup Table/1
  Abs/1 -> 2-D Lookup Table/2
  T/1 -> Abs/1

== system Lib_EMTAT/Components/Power Flow/Three Phase Electric Machine (Sink)/Failure Determination ==
  Fail? : Inport
  Compare To Constant : simulink/Logic and Bit Operations/Compare To Constant  relop===  const=1  OutDataTypeStr=boolean
  Compare To Constant1 : simulink/Logic and Bit Operations/Compare To Constant  relop===  const=2  OutDataTypeStr=boolean
  Data Type Conversion : DataTypeConversion  OutDataTypeStr=double
  Data Type Conversion1 : DataTypeConversion  OutDataTypeStr=double
  Failure Mode : Constant  Value=FM
  Logical Operator : Logic  AllPortsSameDT=off  OutDataTypeStr=boolean
  Logical Operator1 : Logic  AllPortsSameDT=off  OutDataTypeStr=boolean
  OCFail : Outport
  DegFail : Outport  Port=2
  wires:
  Data Type Conversion/1 -> OCFail/1
  Data Type Conversion1/1 -> DegFail/1
  Fail?/1 -> Logical Operator/2, Logical Operator1/2
  Logical Operator1/1 -> Data Type Conversion1/1
  Compare To Constant1/1 -> Logical Operator1/1
  Logical Operator/1 -> Data Type Conversion/1
  Compare To Constant/1 -> Logical Operator/1
  Failure Mode/1 -> Compare To Constant/1, Compare To Constant1/1

== system Lib_EMTAT/Components/Power Flow/Three Phase Electric Machine (Sink)/Open Circuit Failure - Line Current ==
  Failed? : Inport
  I_L_rms : Inport  Port=2
  Constant : Constant  Value=0
  IsInf : RelationalOperator  Operator=isInf  OutDataTypeStr=boolean  RndMeth=Simplest
  IsNaN : RelationalOperator  Operator=isNaN  OutDataTypeStr=boolean  RndMeth=Simplest
  Logical Operator : Logic  Operator=OR  Inputs=3  AllPortsSameDT=off  OutDataTypeStr=boolean
  Switch : Switch  Criteria=u2 > Threshold
  "I_L_rms " : Outport
  wires:
  IsInf/1 -> Logical Operator/3
  IsNaN/1 -> Logical Operator/2
  Logical Operator/1 -> Switch/2
  Switch/1 -> "I_L_rms "/1
  I_L_rms/1 -> Switch/3, IsInf/1, IsNaN/1
  Constant/1 -> Switch/1
  Failed?/1 -> Logical Operator/1

== system Lib_EMTAT/Components/Power Flow/Three Phase Electric Machine (Sink)/Open Circuit Failure - Torque ==
  Failed? : Inport
  T* : Inport  Port=2
  Constant : Constant  Value=0
  IsInf : RelationalOperator  Operator=isInf  OutDataTypeStr=boolean  RndMeth=Simplest
  IsNaN : RelationalOperator  Operator=isNaN  OutDataTypeStr=boolean  RndMeth=Simplest
  Logical Operator : Logic  Operator=OR  Inputs=3  AllPortsSameDT=off  OutDataTypeStr=boolean
  Switch : Switch  Criteria=u2 > Threshold
  "T  " : Outport
  wires:
  Failed?/1 -> Logical Operator/1
  Constant/1 -> Switch/1
  T*/1 -> IsNaN/1, IsInf/1, Switch/3
  Switch/1 -> "T  "/1
  Logical Operator/1 -> Switch/2
  IsNaN/1 -> Logical Operator/2
  IsInf/1 -> Logical Operator/3

== system Lib_EMTAT/Components/Power Flow/Three Phase Electric Machine (Sink)/Open Circuit// Degradation Failure ==
  Eff : Inport
  DegFail? : Inport  Port=2
  OCFail? : Inport  Port=3
  Deg : Inport  Port=4
  Constant : Constant  Value=0
  Constant1 : Constant
  Divide : Product  Inputs=**
  "If degradation failure, penalize Eff." : Switch  Criteria=u2 > Threshold
  "If open circuit failure, set Eff = 0." : Switch  Criteria=u2 > Threshold
  Sum : Sum  Inputs=+-|
  "Eff " : Outport
  wires:
  Sum/1 -> Divide/1
  Constant1/1 -> Sum/1
  Constant/1 -> "If open circuit failure, set Eff = 0."/1
  OCFail?/1 -> "If open circuit failure, set Eff = 0."/2
  "If open circuit failure, set Eff = 0."/1 -> "Eff "/1
  Deg/1 -> Sum/2
  Divide/1 -> "If degradation failure, penalize Eff."/1
  Eff/1 -> "If degradation failure, penalize Eff."/3, Divide/2
  "If degradation failure, penalize Eff."/1 -> "If open circuit failure, set Eff = 0."/3
  DegFail?/1 -> "If degradation failure, penalize Eff."/2

== system Lib_EMTAT/Components/Power Flow/Three Phase Electric Machine (Source)/Compensate for Divide By Zero ==
  note: If Vin is not equal to zero, use its value.
      | If Vin is equal to zero, it will calculate a nan value for Iin. Set Iin to zero.
  PEquivMech : Inport
  N : Inport  Port=2
  Fix Divide By Zero. : Subsystem
  T : Outport
  wires:
  Fix Divide By Zero./1(T) -> T/1
  PEquivMech/1 -> Fix Divide By Zero./2(PEquivMech)
  N/1 -> Fix Divide By Zero./1(N)

== system Lib_EMTAT/Components/Power Flow/Three Phase Electric Machine (Source)/Direction Determination ==
  Eff : Inport
  Pelec : Inport  Port=2
  Divide3 : Product  Inputs=**
  Subsystem : Subsystem
  Switch : Switch  Criteria=u2 > Threshold
  PEquivMech : Outport
  wires:
  Subsystem/1(PEquivMech) -> Switch/3
  Switch/1 -> PEquivMech/1
  Eff/1 -> Divide3/1, Subsystem/2(Eff)
  Divide3/1 -> Switch/1
  Pelec/1 -> Divide3/2, Switch/2, Subsystem/1(Pelec)

== system Lib_EMTAT/Components/Power Flow/Three Phase Electric Machine (Source)/Efficiency ==
  T (lbf-ft) : Inport
  N (RPM) : Inport  Port=2
  2-D Lookup Table : Lookup_n-D  BreakpointsForDimension1=X_C_SpeedVec_M  BreakpointsForDimension2=Y_C_TorqueVec_M  Table=T_C_EffArray_M  ExtrapMethod=Clip  UseLastTableValue=on  InternalRulePriority=Speed  RndMeth=Simplest  InputSameDT=on
      settings: InputPortMap=u0,u1
  Abs : Abs
  Abs1 : Abs
  Saturation : Saturate  UpperLimit=1  LowerLimit=eps
  Eff : Outport
  wires:
  Abs/1 -> 2-D Lookup Table/2
  T (lbf-ft)/1 -> Abs/1
  Saturation/1 -> Eff/1
  2-D Lookup Table/1 -> Saturation/1
  N (RPM)/1 -> Abs1/1
  Abs1/1 -> 2-D Lookup Table/1

== system Lib_EMTAT/Components/Power Flow/Three Phase Electric Machine (Source)/Failure Determination ==
  Fail? : Inport
  Compare To Constant : simulink/Logic and Bit Operations/Compare To Constant  relop===  const=1  OutDataTypeStr=boolean
  Compare To Constant1 : simulink/Logic and Bit Operations/Compare To Constant  relop===  const=2  OutDataTypeStr=boolean
  Data Type Conversion : DataTypeConversion  OutDataTypeStr=double
  Data Type Conversion1 : DataTypeConversion  OutDataTypeStr=double
  Failure Mode : Constant  Value=FM
  Logical Operator : Logic  AllPortsSameDT=off  OutDataTypeStr=boolean
  Logical Operator1 : Logic  AllPortsSameDT=off  OutDataTypeStr=boolean
  OCFail : Outport
  DegFail : Outport  Port=2
  wires:
  Data Type Conversion/1 -> OCFail/1
  Data Type Conversion1/1 -> DegFail/1
  Fail?/1 -> Logical Operator/2, Logical Operator1/2
  Logical Operator1/1 -> Data Type Conversion1/1
  Compare To Constant1/1 -> Logical Operator1/1
  Logical Operator/1 -> Data Type Conversion/1
  Compare To Constant/1 -> Logical Operator/1
  Failure Mode/1 -> Compare To Constant/1, Compare To Constant1/1
